simulink model "Lab4_3"  (R2025a)
settings: Solver=VariableStepAuto  StartTime=0.0  StopTime=27  RelTol=1e-3
settings Model: Creator=andrei  LastModifiedBy=andrei

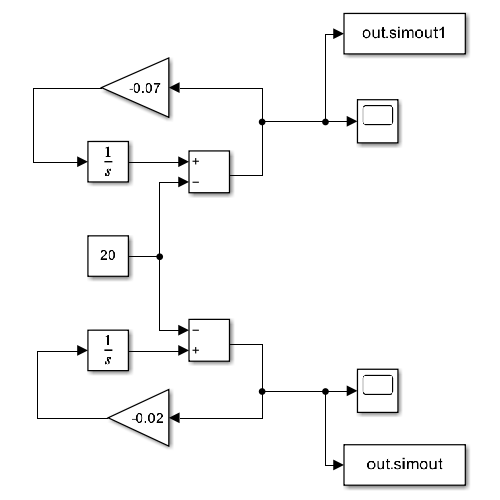
[thumbnail: Simulink's stored preview of the top-level diagram]
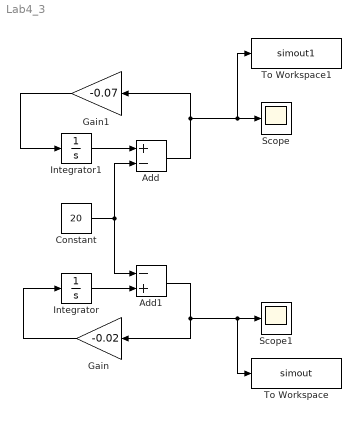
== system Lab4_3 ==
  Add : Sum  Inputs=+-
  Add1 : Sum  Inputs=-+
  Constant : Constant  Value=20
  Gain : Gain  Gain=-0.02
  Gain1 : Gain  Gain=-0.07
  Integrator : Integrator  InitialCondition=130
  Integrator1 : Integrator  InitialCondition=150
  Scope : Scope
      settings: ActiveDisplayYMinimum=-1  ActiveDisplayYMaximum=1
  Scope1 : Scope
  To Workspace : ToWorkspace  VariableName=simout  SaveFormat=Timeseries  SampleTime=-1
  To Workspace1 : ToWorkspace  VariableName=simout1  SaveFormat=Timeseries  SampleTime=-1
  wires:
  Constant/1 -> Add/2, Add1/1
  Integrator1/1 -> Add/1
  Integrator/1 -> Add1/2
  Add/1 -> Scope/1, To Workspace1/1, Gain1/1
  Gain1/1 -> Integrator1/1
  Add1/1 -> To Workspace/1, Scope1/1, Gain/1
  Gain/1 -> Integrator/1
